simulink model "secondSimulation"  (R2020b)
settings: Solver=ode4  StartTime=0.0  StopTime=250.0  FixedStep=0.1227  RelTol=1e-3
libraries: fuzblock x1
settings Model: Creator=sergio  LastModifiedBy=sergio

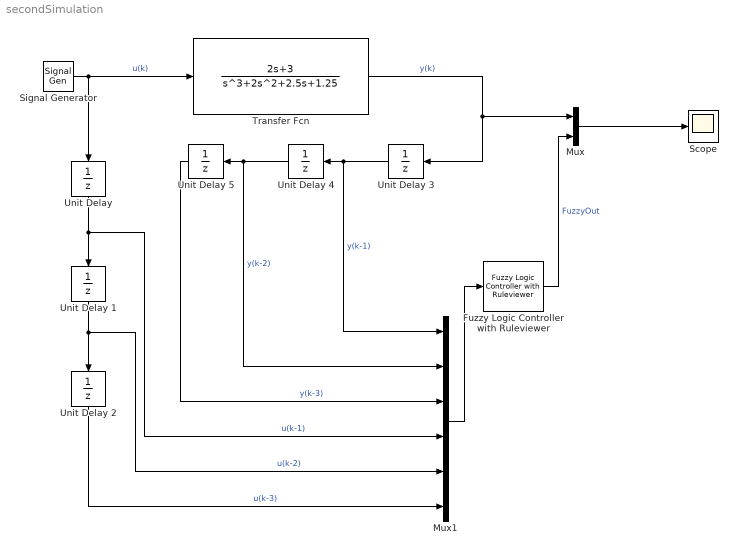
== system secondSimulation ==
  "Fuzzy Logic Controller with Ruleviewer " : fuzblock/Fuzzy Logic  Controller  with Ruleviewer  fismatrix=fuzzySystem  Ts=0.9816
  Mux : Mux  Inputs=2
  Mux1 : Mux  Inputs=6
  "Scope " : Scope
  "Signal Generator " : SignalGenerator  Frequency=0.05  Units=rad/sec
  "Transfer Fcn " : TransferFcn  Numerator=[2 3]  Denominator=[1 2 2.5 1.25]
  Unit Delay {,1..5} (6 alike) : UnitDelay  SampleTime=0.4908  HasFrameUpgradeWarning=on
  wires:
  Unit Delay 4/1 -> Mux1/2, Unit Delay 5/1  "y(k-2)"
  Unit Delay 1/1 -> Unit Delay 2/1, Mux1/5  "u(k-2)"
  Unit Delay 5/1 -> Mux1/3  "y(k-3)"
  Unit Delay 2/1 -> Mux1/6  "u(k-3)"
  "Transfer Fcn "/1 -> Unit Delay 3/1, Mux/1  "y(k)"
  "Unit Delay "/1 -> Unit Delay 1/1, Mux1/4  "u(k-1)"
  Mux/1 -> "Scope "/1
  "Signal Generator "/1 -> "Unit Delay "/1, "Transfer Fcn "/1  "u(k)"
  Unit Delay 3/1 -> Mux1/1, Unit Delay 4/1  "y(k-1)"
  Mux1/1 -> "Fuzzy Logic Controller with Ruleviewer "/1
  "Fuzzy Logic Controller with Ruleviewer "/1 -> Mux/2  "FuzzyOut"
